simulink model "scalar_hw"  (R2023b)
settings: Solver=FixedStepAuto  StartTime=0.0  StopTime=Inf  RelTol=1e-3  EnableMultiTasking=on
values from neighbouring files (symbols this model uses):
  kpp = 3/2 * K^(-2)    (= 1.5)    [init_hw.m]    (also in init_psc_hw.m)
  n = 500    [init_hw.m]    (also in init_psc_hw.m = 300)
  T_pwm = f_clk/(div*f_sw*carr)    (= 9000)    [init_hw.m]    (also in init_psc_hw.m)
  T_s = 1/(2*f_sw)    (= 0.0001)    [init_hw.m]    (also in init_psc_hw.m)
  u_gN = 24    [init_hw.m]    (also in init_psc_hw.m)
  w0_pll = 2*pi*20    (= 125.663706144)    [init_hw.m]    (also in init_psc_hw.m)
  w_b = 0.1*w_N    (= 31.4159265359)    [init_hw.m]    (also in init_psc_hw.m)
  w_N = 2*pi*50    (= 314.159265359)    [init_hw.m]    (also in init_psc_hw.m)
undefined symbols (not defined in the file or in its folder): Down, GPTRIP1SEL, GPTRIP2SEL, TZ1, TZ2, Up
libraries: c2802xlib x13, c2806xlib x4, c280xlib x2, c2000lib x1, simulink x1
(part 2 of 2)

== matlab function scalar_hw/Control block/Scalar control/PWM/MATLAB Function ==
  data: d_abc output double; u_cs_ref input; u_dc input; U_dcmin parameter
function d_abc = PWM(u_cs_ref, u_dc, U_dcmin)

%% Symmetrical suboscillation PWM
% Components of the voltage space vector
u_c_alpha_ref = real(u_cs_ref);
u_c_beta_ref  = imag(u_cs_ref);

% Phase-voltage references
u_ca_ref = u_c_alpha_ref;
u_cb_ref = .5*(-u_c_alpha_ref + sqrt(3)*u_c_beta_ref);
u_cc_ref = .5*(-u_c_alpha_ref - sqrt(3)*u_c_beta_ref);

% Vector of phase-voltage references
u_c_abc_ref = [u_ca_ref; u_cb_ref; u_cc_ref];

% Symmetrization of the references by adding the zero-sequence voltage
u0 = .5*(max(u_c_abc_ref) + min(u_c_abc_ref));
u_c_abc_ref = u_c_abc_ref - u0;

if (u_dc>=U_dcmin)
    % Clipping of the reference voltages such that no phase error is caused. 
    % If all phase voltage reference are realizable (below u_dc/2), m = 1 holds.
    m = max([2.*u_c_abc_ref./u_dc; 1]);
    u_c_abc_ref = u_c_abc_ref./m;
    
    % Duty cycles, which can be directly used for triangle comparison, 
    % if the triangle wave varies between 0...1
    d_abc = .5 + u_c_abc_ref./u_dc;
else
    d_abc = [0; 0; 0];
end

% % Realized voltage vector is calculated from the clamped duty ratios.
% % If the PWM does not saturate, u_c_ref_lim = u_c_ref holds. The realized
% % voltage vector is needed, e.g., for the current-controller antiwindup.
% u_cs_ref_lim = 2/3*(d_abc(1) + d_abc(2)*exp(1j*2*pi/3) ...
%     + d_abc(3)*exp(1j*4*pi/3))*u_dc;
% % In estimated rotor flux coordinates
% u_c_ref_lim = exp(-1j*theta)*u_cs_ref_lim;

== matlab function scalar_hw/Control block/Scalar control/Reference Voltage Limiter/MATLAB Function ==
  data: d_abc input; u_dc input; u_c_ref_lim output; theta input; w_N parameter; T_s parameter
function u_c_ref_lim = ref_lim(d_abc, u_dc, theta, w_N, T_s)

u_c_ref_lim = 0;
% % Realized voltage vector is calculated from the clamped duty ratios.
% % If the PWM does not saturate, u_c_ref_lim = u_c_ref holds. The realized
% % voltage vector is needed, e.g., for the current-controller antiwindup.
u_cs_ref_lim = 2/3*(d_abc(1) + d_abc(2)*exp(1j*2*pi/3) ...
    + d_abc(3)*exp(1j*4*pi/3))*u_dc;

% % In estimated rotor flux coordinates
u_c_ref_lim = exp(-1j*(theta + 1.5 * w_N * T_s)).*u_cs_ref_lim;

== matlab function scalar_hw/Control block/Scalar control/abc to dq transformation ==
  data: i_c output; i_c_abc input; theta input
function i_c = abc2dq(i_c_abc, theta)

% Space Vector Transformation (abc to alpha-beta)
i_cs = 2/3 * (i_c_abc(1) + i_c_abc(2)*exp(1j*2*pi/3) ... 
    + i_c_abc(3)*exp(1j*4*pi/3));

% Coordinate Transformation (Alpha-beta to dq)
i_c = i_cs * exp(-1j*theta);

== matlab function scalar_hw/Control block/MATLAB Function1 ==
  data: u_c input; q_c output; i_c input
function q_c  = fcn(u_c, i_c)

q_c = 3/2*imag((u_c * conj(i_c)));

== matlab function scalar_hw/Control block/Inputs & scaling/MATLAB Function1 ==
  data: i_adc input; i_real output
function i_real = fcn(i_adc)

i_real = -0.0075*i_adc + 15.4645;

== matlab function scalar_hw/Control block/Inputs & scaling/MATLAB Function ==
  data: i_adc input; i_real output
function i_real = fcn(i_adc)

i_real = -0.0075*i_adc + 15.4645;

== matlab function scalar_hw/Control block/Inputs & scaling/MATLAB Function2 ==
  data: i_adc input; i_real output
function i_real = fcn(i_adc)

i_real = -0.0075*i_adc + 15.4645;

== matlab function scalar_hw/Control block/abc to alpha-beta ==
  data: i_alpha output; i_c_abc input; i_beta output
function [i_alpha, i_beta] = abc2alphabeta(i_c_abc)

% Space Vector Transformation (abc to alpha-beta)
i_cs = 2/3 * (i_c_abc(1) + i_c_abc(2)*exp(1j*2*pi/3) ... 
    + i_c_abc(3)*exp(1j*4*pi/3));

i_alpha = real(i_cs);
i_beta = imag(i_cs);

== matlab function scalar_hw/Control block/Inputs & scaling/MATLAB Function9 ==
  data: adc input; y output
function y = fcn(adc)

y = (adc*80/4095-4.067)/1.0114 + 5;

== matlab function scalar_hw/Control block/Inputs & scaling/MATLAB Function4 ==
  data: adc input; y output
function y = fcn(adc)

y = (adc*80/4095-4.067)/1.0114 + 5;

== matlab function scalar_hw/Control block/Inputs & scaling/MATLAB Function3 ==
  data: adc input; y output
function y = fcn(adc)

y = (adc*80/4095-4.067)/1.0114 + 5;

== matlab function scalar_hw/Control block/Inputs & scaling/MATLAB Function5 ==
  data: adc input; y output
function y = fcn(adc)

y = (adc*80/4095-4.067)/1.0114 + 5;

== matlab function scalar_hw/Control block/Inputs & scaling/MATLAB Function6 ==
  data: adc input; y output
function y = fcn(adc)

y = (adc*80/4095-4.067)/1.0114 + 5;
